simulink model "ee5101_5_"  (R2023b)
settings: Solver=VariableStepAuto  StartTime=0.0  StopTime=10.0  RelTol=1e-3
values from neighbouring files (symbols this model uses):
  A = [-8.8487+(a-b)/5  -0.0399  -5.5500+(c+d)/10   3.5846 ... (first row only)    [ee5101_1.m]    (also in ee5101_2.m; ee5101_3.m; ee5101_5.m; ee5103_4.m)
  B = [0.0564+(b/(10+c)) ,0.0319 ... (first row only)    [ee5101_1.m]    (also in ee5101_2.m; ee5101_3.m; ee5101_5.m; ee5103_4.m)
  C = [-3.2988, -2.1932+(10*c +d)/(100+5*a) ,0.0370 ,-0.0109 ... (first row only)    [ee5101_1.m]    (also in ee5101_2.m; ee5101_3.m; ee5101_5.m; ee5103_4.m)
  H = H_1'    [ee5101_5.m]
  k1 = K1(:,1:4)    [ee5101_5.m]
  k2 = K1(:,5:6)    [ee5101_5.m]
settings Model: Creator=perrymiao  LastModifiedBy=perrymiao

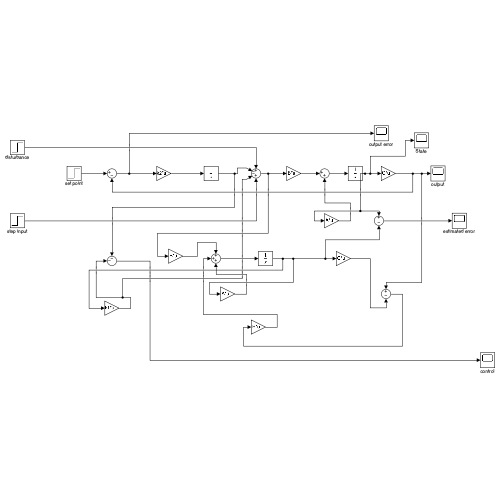
[thumbnail: Simulink's stored preview of the top-level diagram]
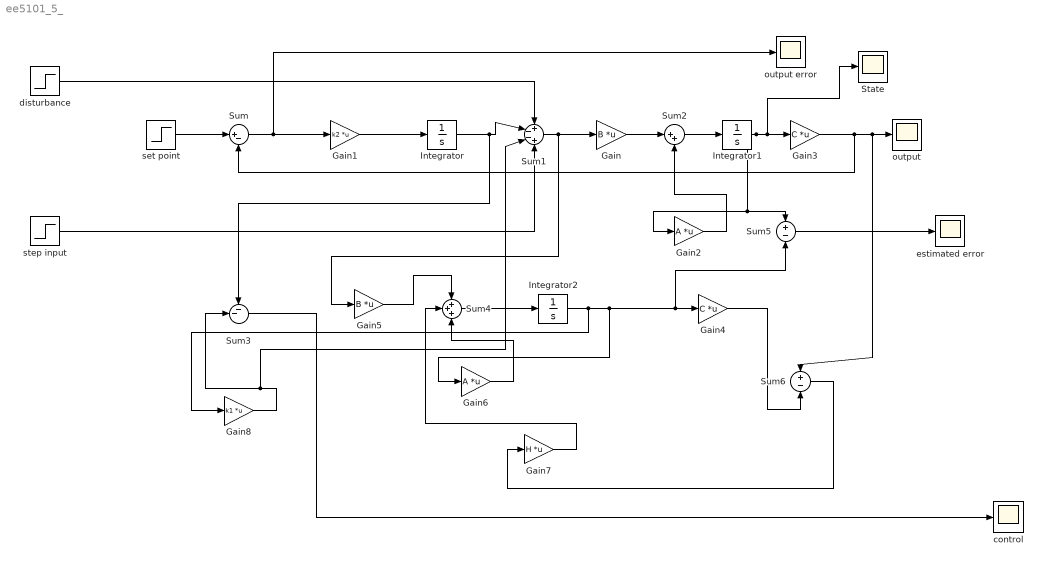
== system ee5101_5_ ==
  Gain : Gain  Gain=B  Multiplication=Matrix(K*u)
  Gain1 : Gain  Gain=k2  Multiplication=Matrix(K*u)
  Gain2 : Gain  Gain=A  Multiplication=Matrix(K*u)
  Gain3 : Gain  Gain=C  Multiplication=Matrix(K*u)
  Gain4 : Gain  Gain=C  Multiplication=Matrix(K*u)
  Gain5 : Gain  Gain=B  Multiplication=Matrix(K*u)
  Gain6 : Gain  Gain=A  Multiplication=Matrix(K*u)
  Gain7 : Gain  Gain=H  Multiplication=Matrix(K*u)
  Gain8 : Gain  Gain=k1  Multiplication=Matrix(K*u)
  Integrator : Integrator
  Integrator1 : Integrator
  Integrator2 : Integrator
  State : Scope
  Sum : Sum  Inputs=|+-
  Sum1 : Sum  Inputs=+--+
  Sum2 : Sum  Inputs=|++
  Sum3 : Sum  Inputs=--|
  Sum4 : Sum  Inputs=+++
  Sum5 : Sum  Inputs=+-
  Sum6 : Sum  Inputs=+-
  control : Scope
  disturbance : Step  Time=0  Before=[0 0]'  After=[0 1]'  SampleTime=0
  estimated error : Scope
  output : Scope
  output error : Scope
  set point : Step  Time=0  Before=[0 0]'  After=[0 1]'  SampleTime=0  VectorParams1D=off
  step input : Step  Time=0  Before=[0 0]'  After=[0 1]'  SampleTime=0  VectorParams1D=off
  wires:
  Sum/1 -> output error/1, Gain1/1
  set point/1 -> Sum/1
  Gain1/1 -> Integrator/1
  Integrator/1 -> Sum3/1, Sum1/2
  Sum1/1 -> Gain5/1, Gain/1
  Gain/1 -> Sum2/1
  Sum2/1 -> Integrator1/1
  disturbance/1 -> Sum1/1
  step input/1 -> Sum1/4
  Gain3/1 -> Sum/2, Sum6/1, output/1
  Integrator1/1 -> State/1, Gain3/1, Sum5/1, Gain2/1
  Gain2/1 -> Sum2/2
  Sum5/1 -> estimated error/1
  Integrator2/1 -> Gain8/1, Gain6/1, Sum5/2, Gain4/1
  Gain4/1 -> Sum6/2
  Sum4/1 -> Integrator2/1
  Gain5/1 -> Sum4/1
  Gain6/1 -> Sum4/3
  Gain7/1 -> Sum4/2
  Sum6/1 -> Gain7/1
  Gain8/1 -> Sum1/3, Sum3/2
  Sum3/1 -> control/1
